simulink model "fbg_filtered (1)"  (R2023b)
settings: Solver=VariableStepAuto  StartTime=0.0  StopTime=10.0  RelTol=1e-3
libraries: simulink x1
settings Model: Creator=user  LastModifiedBy=user

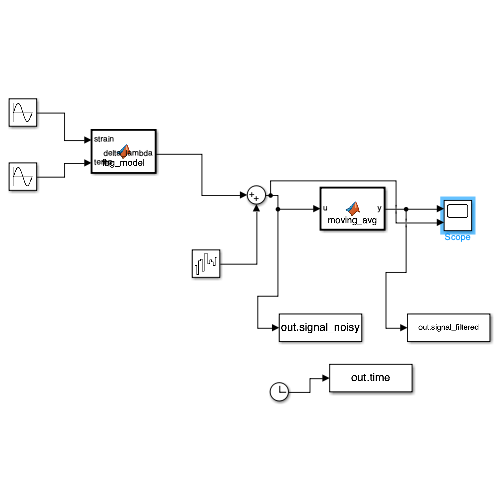
[thumbnail: Simulink's stored preview of the top-level diagram]
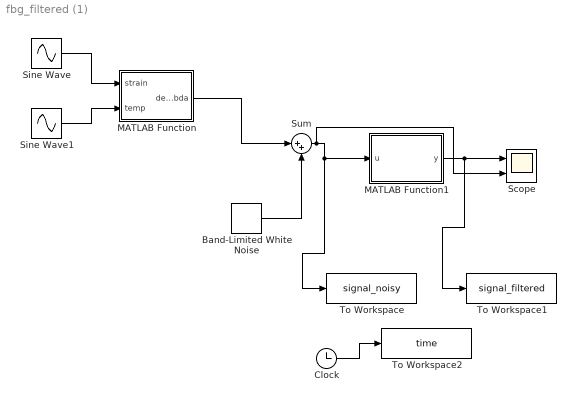
== system fbg_filtered (1) ==
  Band-Limited White Noise : simulink/Sources/Band-Limited White Noise  Cov=[0.1]  Ts=0.1  seed=[23341]
  Clock : Clock
      settings: Decimation=2
  MATLAB Function : MATLAB Function  TreatAsAtomicUnit=on
  MATLAB Function1 : MATLAB Function  TreatAsAtomicUnit=on
  Scope : Scope  NumInputPorts=2
  Sine Wave : Sin  Amplitude=0.005  Bias=0.003  SampleTime=0
  Sine Wave1 : Sin  Amplitude=10  Bias=30  SampleTime=0
  Sum : Sum  Inputs=|++
  To Workspace : ToWorkspace  VariableName=signal_noisy  SampleTime=-1
  To Workspace1 : ToWorkspace  VariableName=signal_filtered  SampleTime=-1
  To Workspace2 : ToWorkspace  VariableName=time  SaveFormat=Timeseries  SampleTime=-1
  wires:
  Sine Wave/1 -> MATLAB Function/1(strain)
  Sine Wave1/1 -> MATLAB Function/2(temp)
  MATLAB Function/1(delta_lambda) -> Sum/1
  Band-Limited White Noise/1 -> Sum/2
  Clock/1 -> To Workspace2/1
  MATLAB Function1/1(y) -> To Workspace1/1, Scope/1
  Sum/1 -> Scope/2, MATLAB Function1/1(u), To Workspace/1

== matlab function fbg_filtered (1)/MATLAB Function ==
  data: strain input; delta_lambda output; temp input
function delta_lambda = fbg_model(strain, temp)

lambda_B = 1550;
pe = 0.22;
T0 = 25;
k = 1e-6;

delta_lambda = lambda_B*(1-pe)*strain + lambda_B*k*(temp - T0);

== matlab function fbg_filtered (1)/MATLAB Function1 ==
  data: u input; y output
function y = moving_avg(u)

persistent buffer
N = 10;

if isempty(buffer)
    buffer = zeros(1,N);
end

buffer = [buffer(2:end) u];
y = mean(buffer);
